simulink model "MotorDriveUnitBasic_test_harness"  (R2020b)
settings: Solver=daessc  StartTime=0.0  StopTime=t_end  RelTol=1e-3  AbsTol=1e-3
PreLoadFcn:
  | MotorDriveUnitBasic_setup
undefined symbols (not defined in the file or in its folder): Minus, Plus
libraries: fl_lib x4, nesl_utility x2, EVComponents_utility_lib x1
settings Model: Creator=isaacito  LastModifiedBy=isaacito
settings SolverCC: AutoScaleAbsTol=off
settings DataIOCC: DSMLogging=off
settings DebuggingCC: SymbolicDimsDataTypeCodeGenerationDiagnostic=none
settings SFSimCC: CustomCodeUndefinedFunction=UseInterfaceOnly
settings SimscapeCC: SimscapeLogType=all  SimscapeLogSimulationStatistics=on  SimscapeLogLimitData=off  SimscapeLogDataHistory=10000

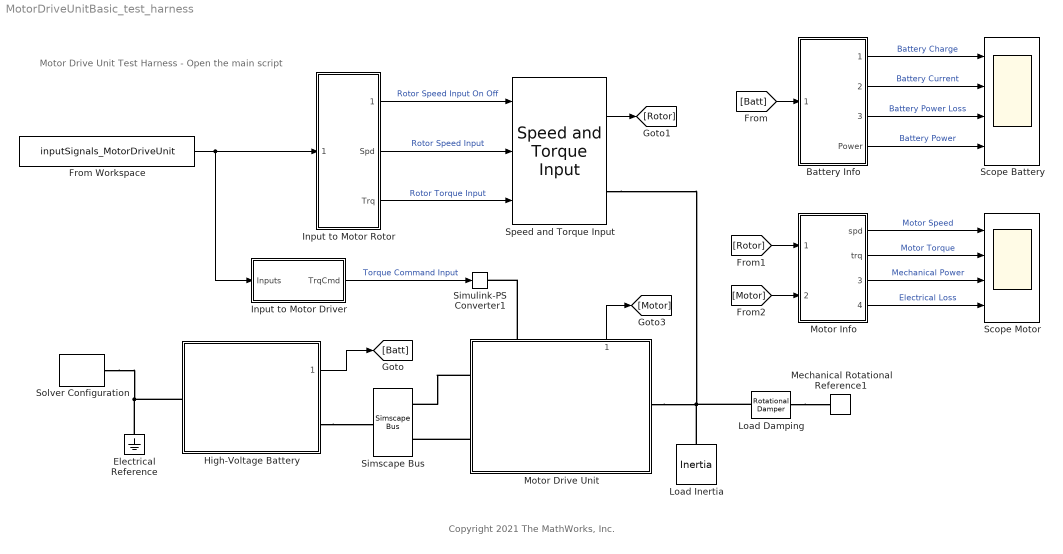
== system MotorDriveUnitBasic_test_harness ==
  note: Motor Drive Unit Test Harness
      | - Open the main script
  note: Copyright 2021 The MathWorks, Inc.
  Battery Info : Subsystem
  Electrical Reference : fl_lib/Electrical/Electrical Elements/Electrical Reference
  From Workspace : FromWorkspace  VariableName=inputSignals_MotorDriveUnit  OutDataTypeStr=Bus: inputBus_MotorDriveUnit  Interpolate=off  OutputAfterFinalValue=Holding final value
      settings: AttributesFormatString=%<OutDataTypeStr>
  High-Voltage Battery : Subsystem  ReferencedSubsystem=BatteryHVBasic_refsub
  Input to Motor Driver : Subsystem
  Input to Motor Rotor : Subsystem
  Load Damping : fl_lib/Mechanical/Rotational Elements/Rotational Damper  D=0.01 m*N/rpm  w_specify=off  w_priority=None  w=0 rad/s  w_nominal_specify=off  w_nominal_unit=rad/s  w_nominal_value=1  t_specify=off  t_priority=None  t=0 N*m  t_nominal_specify=off  t_nominal_unit=N*m  t_nominal_value=1
  Load Inertia : fl_lib/Mechanical/Rotational Elements/Inertia  inertia=0.05 kg*m^2  num_ports=foundation.enum.numPorts2.one  w_specify=off  w_priority=High  w=0 rad/s  w_nominal_specify=off  w_nominal_unit=rad/s  w_nominal_value=1  t_specify=off  t_priority=None  t=0 N*m  t_nominal_specify=off  t_nominal_unit=N*m  t_nominal_value=1
  Mechanical Rotational Reference1 : fl_lib/Mechanical/Rotational Elements/Mechanical Rotational Reference
  Motor Drive Unit : Subsystem  ReferencedSubsystem=MotorDriveUnitBasic_refsub
      settings: PortSchema="{\"entries\":[{\"content\":{\"sides\":[{\"content\":{\"connectorIds\":[\"LConn1\",\"LConn2\"]},\"type\":\"ConnectorPlacement.EquallySpacedRectSide\",\"uuid\":\"e655f04c-0831-4715-9239-c12e978aab5b\"},{\"content\":{\"connectorIds\":[\"RConn1\"],\"side\":\"RIGHT\"},\"type\":\"ConnectorPlacement.EquallySpacedRectSide\",\"uuid\":\"e54f9812-1fa1-41d5-85ff-8aa3e8117d91\"},{\"content\":{\"connectorIds\":[\"LConn3\",\"Out1\"],\"side\":\"TOP\"},\"type\":\"ConnectorPlacement.EquallySpacedRectSide\",\"uuid\":\"53d3fec0-b122-47d6-942d-255744ffbc1f\"},{\"content\":{\"connectorIds\":[],\"side\":\"HIDDEN\"},\"type\":\"ConnectorPlacement.EquallySpacedRectSide\",\"uuid\":\"2a8d4fa9-f44a-44a1-a9cb-45b1b6dc3be9\"}]},\"type\":\"ConnectorPlacement.EquallySpacedConnector\",\"uuid\":\"9d4c78d8-e120-4f49-8bbf-58b9e828fd7c\"}],\"packageUris\":[\"http://schema.mathworks.com/mf0/Connector/R2020b\"],\"version\":\"1.0\"}"
  Motor Info : Subsystem
  Scope Battery : Scope  NumInputPorts=4
  Scope Motor : Scope  NumInputPorts=4
  Simscape Bus : SimscapeBus  HierarchyStrings=Plus;Minus
  Simulink-PS Converter1 : nesl_utility/Simulink-PS Converter  PhysicalDomain=network_engine_domain  SubClassName=ps_input  LeftPortType=input  RightPortType=output  PseudoPeriodic=off  Frequencies=[]  NoiseDistribution=none  NoiseParameters=[]  Unit=N*m  AffineConversion=off  FilteringAndDerivatives=provide  SimscapeFilterOrder=1  InputFilterTimeConstant=0.001  UdotUserProvided=0
      settings: SourceProductName=Utilities
  Solver Configuration : nesl_utility/Solver Configuration  PhysicalDomain=network_engine_domain  SubClassName=solver  LeftPortType=input  RightPortType=generic  Tones=[]  Harmonics=[]  SimulateNoise=off  Profile=off  UseLocalSampling=off  EnableSwitchedLinearOptims=on  FrequencyDomain=off  UseCCode=off  RelTol=0.001  AbsTol=1e-06  MinStep=1e-09  ToWorkspace=off  RevertToSquareIcSolve=off  NumHomotopyIterations=100  PhasorMode=off  PhasorModeNumHarmonics=1  DoDC=off  ResidualTolerance=1e-09  UseLocalSolver=off  LocalSolverChoice=NE_BACKWARD_EULER_ADVANCER  LocalSolverSampleTime=0.001  DoFixedCost=off  MaxNonlinIter=3  MaxModeIter=2  ComputeImpulses=off  ImpulseIterations=2  LinearAlgebra=auto  EquationFormulation=NE_TIME_EF  DelaysMemoryBudget=1024  AutomaticFiltering=on  FilteringTimeConstant=0.001  PartitionStorageMethod=AS_NEEDED  PartitionMemoryBudget=1024  PartitionMethod=ROBUST
      settings: SourceProductName=Utilities
  Speed and Torque Input : EVComponents_utility_lib/Speed and Torque Input  t_friction=10000  t_locked=10000  w_tol=0.001  initial_state_locked=sdl.enum.initial_lock.unlocked
  wires:
  Speed and Torque Input/1 -> [Rotor]
  [Rotor] -> Motor Info/1(RotorInfo)
  Motor Info/1(spd) -> Scope Motor/1  "Motor Speed"
  Input to Motor Rotor/1(Spd_OnOff) -> Speed and Torque Input/1  "Rotor Speed Input On Off"
  Input to Motor Rotor/2(Spd) -> Speed and Torque Input/2  "Rotor Speed Input"
  Input to Motor Rotor/3(Trq) -> Speed and Torque Input/3  "Rotor Torque Input"
  Input to Motor Driver/1(TrqCmd) -> Simulink-PS Converter1/1  "Torque Command Input"
  [Batt] -> Battery Info/1(BattInfo)
  Battery Info/1(Charge) -> Scope Battery/1  "Battery Charge"
  Battery Info/2(Current) -> Scope Battery/2  "Battery Current"
  Battery Info/3(PowerLoss) -> Scope Battery/3  "Battery Power Loss"
  Battery Info/4(Power) -> Scope Battery/4  "Battery Power"
  Motor Info/2(trq) -> Scope Motor/2  "Motor Torque"
  Motor Drive Unit/1 -> [Motor]
  [Motor] -> Motor Info/2(MotorInfo)
  From Workspace/1 -> Input to Motor Driver/1(Inputs), Input to Motor Rotor/1(Inputs)
  Motor Info/3(mech_pow) -> Scope Motor/3  "Mechanical Power"
  Motor Info/4(elec_loss) -> Scope Motor/4  "Electrical Loss"
  High-Voltage Battery/1 -> [Batt]
  connections:
  Electrical Reference/LConn1 -- High-Voltage Battery/LConn1 -- Solver Configuration/RConn1
  Load Inertia/LConn1 -- Speed and Torque Input/RConn1 -- Motor Drive Unit/RConn1 -- Load Damping/LConn1
  Load Damping/RConn1 -- Mechanical Rotational Reference1/LConn1
  Motor Drive Unit/LConn3 -- Simulink-PS Converter1/RConn1
  Motor Drive Unit/LConn1 -- Simscape Bus/LConn1
  Motor Drive Unit/LConn2 -- Simscape Bus/LConn2
  High-Voltage Battery/RConn1 -- Simscape Bus/RConn1

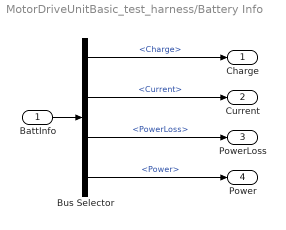
== system MotorDriveUnitBasic_test_harness/Battery Info ==
  BattInfo : Inport
  Bus Selector : BusSelector  OutputSignals=Charge,Current,PowerLoss,Power
  Charge : Outport
  Current : Outport  Port=2
  PowerLoss : Outport  Port=3
  Power : Outport  Port=4
  wires:
  Bus Selector/1 -> Charge/1  "<Charge>"
  BattInfo/1 -> Bus Selector/1
  Bus Selector/3 -> PowerLoss/1  "<PowerLoss>"
  Bus Selector/4 -> Power/1  "<Power>"
  Bus Selector/2 -> Current/1  "<Current>"

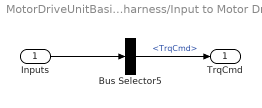
== system MotorDriveUnitBasic_test_harness/Input to Motor Driver ==
  Inputs : Inport
  Bus Selector5 : BusSelector  OutputSignals=TrqCmd
  TrqCmd : Outport
  wires:
  Bus Selector5/1 -> TrqCmd/1  "<TrqCmd>"
  Inputs/1 -> Bus Selector5/1

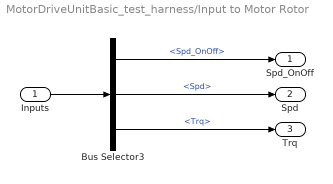
== system MotorDriveUnitBasic_test_harness/Input to Motor Rotor ==
  Inputs : Inport
  Bus Selector3 : BusSelector  OutputSignals=Spd_OnOff,Spd,Trq
  Spd_OnOff : Outport
  Spd : Outport  Port=2
  Trq : Outport  Port=3
  wires:
  Bus Selector3/2 -> Spd/1  "<Spd>"
  Inputs/1 -> Bus Selector3/1
  Bus Selector3/1 -> Spd_OnOff/1  "<Spd_OnOff>"
  Bus Selector3/3 -> Trq/1  "<Trq>"

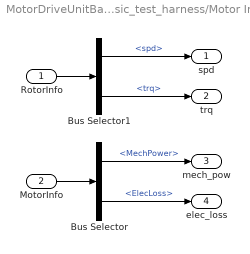
== system MotorDriveUnitBasic_test_harness/Motor Info ==
  RotorInfo : Inport
  MotorInfo : Inport  Port=2
  Bus Selector : BusSelector  OutputSignals=MechPower,ElecLoss
  Bus Selector1 : BusSelector  OutputSignals=spd,trq
  spd : Outport
  trq : Outport  Port=2
  mech_pow : Outport  Port=3
  elec_loss : Outport  Port=4
  wires:
  RotorInfo/1 -> Bus Selector1/1
  Bus Selector1/1 -> spd/1  "<spd>"
  Bus Selector1/2 -> trq/1  "<trq>"
  MotorInfo/1 -> Bus Selector/1
  Bus Selector/2 -> elec_loss/1  "<ElecLoss>"
  Bus Selector/1 -> mech_pow/1  "<MechPower>"
